simulink library "EV_VLD"  (R2019b)
settings: Solver=VariableStepAuto  StartTime=0.0  StopTime=10.0  RelTol=1e-3
undefined symbols (not defined in the file): DiscIntNeverNeededParam
libraries: $bdroot x2, simulink x2
(part 1 of 2)
Description:
  | User defined library for EV
settings Model: Creator=francesco.mantuano  LastModifiedBy=francesco.mantuano

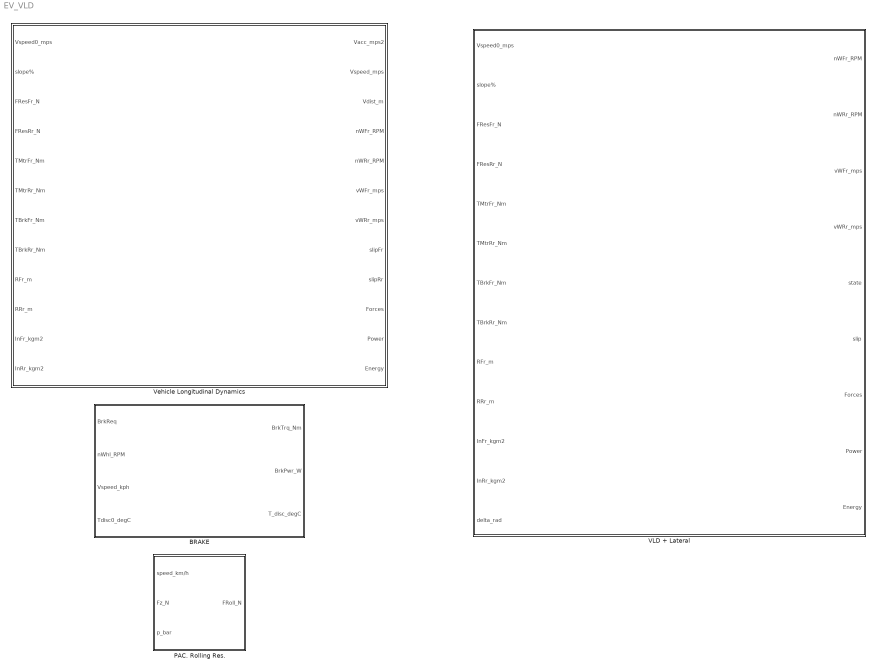
== system EV_VLD ==
  BRAKE : Subsystem  mask(Brake){MxTrq_Nm=7200, eff=1, HC_disc=3420, T_env_degC=0, R_StoC_KpW=0.0035*0.8, HTC_v_bp=0:150:300, HTC_map=[3 20 40]}
      mask prompts: MxTrq_Nm "Max torque [Nm]"; eff "Efficiency"; HC_disc "HC_disc [J/K]"; T_env_degC "T_env [°C]"; R_StoC_KpW "R_StoC [K/W]"; HTC_v_bp "Speed [km/h] bp"; HTC_map "HTC [W/K]"
      mask help: The BRAKE block gives as outputs the brake torque and the thrmal power dissipated. It also estimates the brake discs temperature.
      mask DialogControl Container2 Prompt: Inputs description
      mask DialogControl DescTextVar Prompt: - BrkReq: brake requested from VCU (0 < BrkReq < 1) [-]
      mask DialogControl Control4 Prompt: - nWhl_RPM: wheels speed [RPM]
      mask DialogControl Control5 Prompt: - Vspeed_mps: vehicle speed [m/s]
      mask DialogControl Control6 Prompt: - Tbrake0_degC: initial temperature of the brake discs [°C]
      mask DialogControl Container3 Prompt: Parameters
      mask DialogControl Container9 Prompt: Mechanical
      mask DialogControl Container5 Prompt: Thermal
      mask DialogControl Container10 Prompt: HTC map
  PAC. Rolling Res. : Subsystem  mask(Rolling Resistance (Pacejka)){Vref_kmph=130, Fzref_N=5540, pref_bar=3, SF=1.15, qsy1=8.37e-3, qsy2=0, qsy3=1.02e-3, qsy4=-2.51e-5, qsy5=0, qsy6=0, qsy7=0.865, qsy8=-0.337}
      mask prompts: Vref_kmph "Vref [km/h]"; Fzref_N "Fzref [N]"; pref_bar "pref [bar]"; SF "scaling factor"
      mask help: Pacejka rolling resistance force calculation (one tire)
  VLD + Lateral : Subsystem  mask(Vehicle Longitudinal Dynamics){mass_kg=2000, J_kgm2=3000, WDFr_p=48, l_m=2.800, t1=1.765, t2=1.725, hCOG_m=0.45, h1=0.15, h2=0.18, q=0.285, k1=1e5, k2=1.2e5, Tenv_degC=23, Fsurf_sm=2.4, Cl_Fr1=0, Cl_Rr1=0, Cd1=0.35, WRS_kmph=160, Cl_Fr2=-0.1, Cl_Rr2=-0.2, Cd2=0.4, VLoad_bp=0, slip_bp=0, frictionFr_map=0, frictionRr_map=0, VLoada_bp=0, slipa_bp=0, FyFr_map=0, FyRr_map=0}
      mask prompts: mass_kg "Mass [kg]"; J_kgm2 "Yaw Inertia [kg*sm]"; WDFr_p "Weight distribution Front [%]"; l_m "Vehicle wheelbase [m]"; t1 "Front track [m]"; t2 "Rear track [m]"; hCOG_m "COG height [m]"; h1 "Front Roll center height [m]"; h2 "Rear Roll center height [m]"; q "COG-RollAxle distance [m]"; k1 "Front Roll stiffness [Nm/rad]"; k2 "Rear Roll stiffness [Nm/rad]"; Tenv_degC "Ambient temperature [degC]"; Fsurf_sm "Frontal area [sm]"; Cl_Fr1 "Lift coefficient FRONT"; Cl_Rr1 "Lift coefficient REAR"; Cd1 "Drag coefficient"; WRS_kmph "Wing Raise Speed [km/h]"; Cl_Fr2 "Lift coefficient FRONT"; Cl_Rr2 "Lift coefficient REAR"; Cd2 "Drag coefficient"; VLoad_bp "Vertical Load [N] breakpoints"; slip_bp "longitudinal slip [-] breakpoints"; frictionFr_map "Front friction coefficient MAP"; frictionRr_map "Rear friction coefficient MAP"; VLoada_bp "Vertical Load [N] breakpoints"; slipa_bp "lateral slip [rad] breakpoints"; FyFr_map "Front friction coefficient MAP"; FyRr_map "Rear friction coefficient MAP"
      mask help:
      | The VLD block is an estimation block that calculate the Vehicle state. It also outputs the Forces, the Power and the Energy involved.
      | NOTE THAT: the motor torque is already delayed in the estimation block.
      mask DialogControl Container2 Prompt: Inputs description
      mask DialogControl DescTextVar Prompt: - Vspeed0_mps: initial speed of the vehicle [m/s]
      mask DialogControl Control4 Prompt: - slope%: inclination of the road [%]
      mask DialogControl Control5 Prompt: - FResFr_N: front resistance force acting before the tires [N]
      mask DialogControl Control6 Prompt: - FResRr_N: rear resistance force acting before the tires [N]
      mask DialogControl Control8 Prompt: - TMtrFr_Nm: front motor torque [Nm]
      mask DialogControl Control9 Prompt: - TMtrRr_Nm: rear motor torque [Nm]
      mask DialogControl Control10 Prompt: - TBrkFr_Nm: front brake torque [Nm]
      mask DialogControl Control11 Prompt: - TBrkRr_Nm: rear brake torque [Nm]
      mask DialogControl Control12 Prompt: - RFr_m: front rolling radius [m]
      mask DialogControl Control13 Prompt: - RRr_m: rear rolling radius [m]
      mask DialogControl Control14 Prompt: - InFr_kgm2: front rotational inertia [kg*sm]
      mask DialogControl Control15 Prompt: - InRr_kgm2: rear rotational inertia [kg*sm]
      mask DialogControl Container11 Prompt: Outputs description
      mask DialogControl Control16 Prompt: - Vacc_mps2: vehicle acceleration [m/s2]
      mask DialogControl Control17 Prompt: - Vspeed_mps: vehicle speed [m/s]
      mask DialogControl Control18 Prompt: - Vdist_m: distance traveled [m]
      mask DialogControl Control19 Prompt: - nWFr_RPM: front wheels RPM
      mask DialogControl Control20 Prompt: - nWRr_RPM: rear wheels RPM
      mask DialogControl Control21 Prompt: - vWFr_mps: front wheels speed [m/s]
      mask DialogControl Control22 Prompt: - vWRr_mps: rear wheels speed [m/s]
      mask DialogControl Control23 Prompt: - slipFr: front tires longitudinal slip [-]
      mask DialogControl Control24 Prompt: - slipRr: rear tires longitudinal slip [-]
      mask DialogControl Container12 Prompt: Forces
      mask DialogControl Control25 Prompt: - mequiv_kg: vehicle equivalent mass [kg]
      mask DialogControl Control26 Prompt: - WFr_N: front vertical load [N]
      mask DialogControl Control27 Prompt: - WRr_N: rear vertical load [N]
      mask DialogControl Control28 Prompt: - FWhl_N: total traction force (includes braking force) [N]
      mask DialogControl Control29 Prompt: - FResTot_N: total resistance force [N]
      mask DialogControl Control30 Prompt: - FTot_N: FWhl - FResTot [N]
      mask DialogControl Container14 Prompt: Power
      mask DialogControl Control31 Prompt: - PWhl_W: traction power (includes brake) at wheels [W]
      mask DialogControl Control32 Prompt: - PWhlMtr_W: motor traction power at wheels [W]
      mask DialogControl Container13 Prompt: Energy
      mask DialogControl Control33 Prompt: - EWhlMtrC_kWh: motor charge energy at wheels [kWh]
      mask DialogControl Control34 Prompt: - EWhlMtrD_kWh: motor discharge energy at wheels [kWh]
      mask DialogControl Control35 Prompt: - EDrag_kWh: drag energy loss [kWh]
      mask DialogControl Container3 Prompt: Vehicle parameters
      mask DialogControl Container9 Prompt: Weights
      mask DialogControl Container5_copy Prompt: Aerodynamics
      mask DialogControl Container10 Prompt: Active Wing
      mask DialogControl Container5 Prompt: Tire
      mask DialogControl Container17 Prompt: Longitudinal
      mask DialogControl Container17_copy Prompt: Lateral
  Vehicle Longitudinal Dynamics : Subsystem  mask(Vehicle Longitudinal Dynamics){slip=0, mass_kg=2000, WDFr_p=48, l_m=2.800, hCOG_m=0.45, tow_mass_kg=0, h_tow=0.5, Tenv_degC=23, Fsurf_sm=2.4, Cl_Fr1=0, Cl_Rr1=0, Cd1=0, WRS_kmph=0, Cl_Fr2=0, Cl_Rr2=0, Cd2=0, VLoad_bp=zeros(1,2), slip_bp=zeros(1,2), frictionFr_map=zeros(2,2), frictionRr_map=zeros(2,2), mu_front=0.8, mu_rear=0.8}
      mask prompts: slip "slip (== 1 slip model, == 0 no-slip model)"; mass_kg "Mass [kg]"; WDFr_p "Weight distribution Front [%]"; l_m "Vehicle wheelbase [m]"; hCOG_m "COG height [m]"; tow_mass_kg "Mass [kg]"; h_tow "Hitch height [m]"; Tenv_degC "Ambient temperature [degC]"; Fsurf_sm "Frontal area [sm]"; Cl_Fr1 "Lift coefficient FRONT"; Cl_Rr1 "Lift coefficient REAR"; Cd1 "Drag coefficient"; WRS_kmph "Wing Raise Speed [km/h]"; Cl_Fr2 "Lift coefficient FRONT"; Cl_Rr2 "Lift coefficient REAR"; Cd2 "Drag coefficient"; VLoad_bp "Vertical Load [N] breakpoints"; slip_bp "longitudinal slip [-] breakpoints"; frictionFr_map "Front friction coefficient MAP"; frictionRr_map "Rear friction coefficient MAP"; mu_front "front mu [-]"; mu_rear "rear mu [-]"
      mask help:
      | The VLD block is an estimation block that calculate the Vehicle state. It also outputs the Forces, the Power and the Energy involved.
      | NOTE THAT: the motor torque is already delayed in the estimation block.
      mask DialogControl Container2 Prompt: Inputs description
      mask DialogControl DescTextVar Prompt: - Vspeed0_mps: initial speed of the vehicle [m/s]
      mask DialogControl Control4 Prompt: - slope%: inclination of the road [%]
      mask DialogControl Control5 Prompt: - FResFr_N: front resistance force acting before the tires [N]
      mask DialogControl Control6 Prompt: - FResRr_N: rear resistance force acting before the tires [N]
      mask DialogControl Control8 Prompt: - TMtrFr_Nm: front motor torque [Nm]
      mask DialogControl Control9 Prompt: - TMtrRr_Nm: rear motor torque [Nm]
      mask DialogControl Control10 Prompt: - TBrkFr_Nm: front brake torque [Nm]
      mask DialogControl Control11 Prompt: - TBrkRr_Nm: rear brake torque [Nm]
      mask DialogControl Control12 Prompt: - RFr_m: front rolling radius [m]
      mask DialogControl Control13 Prompt: - RRr_m: rear rolling radius [m]
      mask DialogControl Control14 Prompt: - InFr_kgm2: front rotational inertia [kg*sm]
      mask DialogControl Control15 Prompt: - InRr_kgm2: rear rotational inertia [kg*sm]
      mask DialogControl Container11 Prompt: Outputs description
      mask DialogControl Control16 Prompt: - Vacc_mps2: vehicle acceleration [m/s2]
      mask DialogControl Control17 Prompt: - Vspeed_mps: vehicle speed [m/s]
      mask DialogControl Control18 Prompt: - Vdist_m: distance traveled [m]
      mask DialogControl Control19 Prompt: - nWFr_RPM: front wheels RPM
      mask DialogControl Control20 Prompt: - nWRr_RPM: rear wheels RPM
      mask DialogControl Control21 Prompt: - vWFr_mps: front wheels speed [m/s]
      mask DialogControl Control22 Prompt: - vWRr_mps: rear wheels speed [m/s]
      mask DialogControl Control23 Prompt: - slipFr: front tires longitudinal slip [-]
      mask DialogControl Control24 Prompt: - slipRr: rear tires longitudinal slip [-]
      mask DialogControl Container12 Prompt: Forces
      mask DialogControl Control25 Prompt: - mequiv_kg: vehicle equivalent mass [kg]
      mask DialogControl Control26 Prompt: - WFr_N: front vertical load [N]
      mask DialogControl Control27 Prompt: - WRr_N: rear vertical load [N]
      mask DialogControl Control28 Prompt: - FWhl_N: total traction force (includes braking force) [N]
      mask DialogControl Control29 Prompt: - FResTot_N: total resistance force [N]
      mask DialogControl Control30 Prompt: - FTot_N: FWhl - FResTot [N]
      mask DialogControl Container14 Prompt: Power
      mask DialogControl Control31 Prompt: - PWhl_W: traction power (includes brake) at wheels [W]
      mask DialogControl Control32 Prompt: - PWhlMtr_W: motor traction power at wheels [W]
      mask DialogControl Container13 Prompt: Energy
      mask DialogControl Control33 Prompt: - EWhlMtrC_kWh: motor charge energy at wheels [kWh]
      mask DialogControl Control34 Prompt: - EWhlMtrD_kWh: motor discharge energy at wheels [kWh]
      mask DialogControl Control35 Prompt: - EDrag_kWh: drag energy loss [kWh]
      mask DialogControl Container3 Prompt: Vehicle parameters
      mask DialogControl Container9 Prompt: Weights
      mask DialogControl Container19 Prompt: Towing
      mask DialogControl Container5_copy Prompt: Aerodynamics
      mask DialogControl Container10 Prompt: Active Wing
      mask DialogControl Container5 Prompt: Tire
      mask DialogControl Container17 Prompt: slip model
      mask DialogControl Container18 Prompt: no-slip model

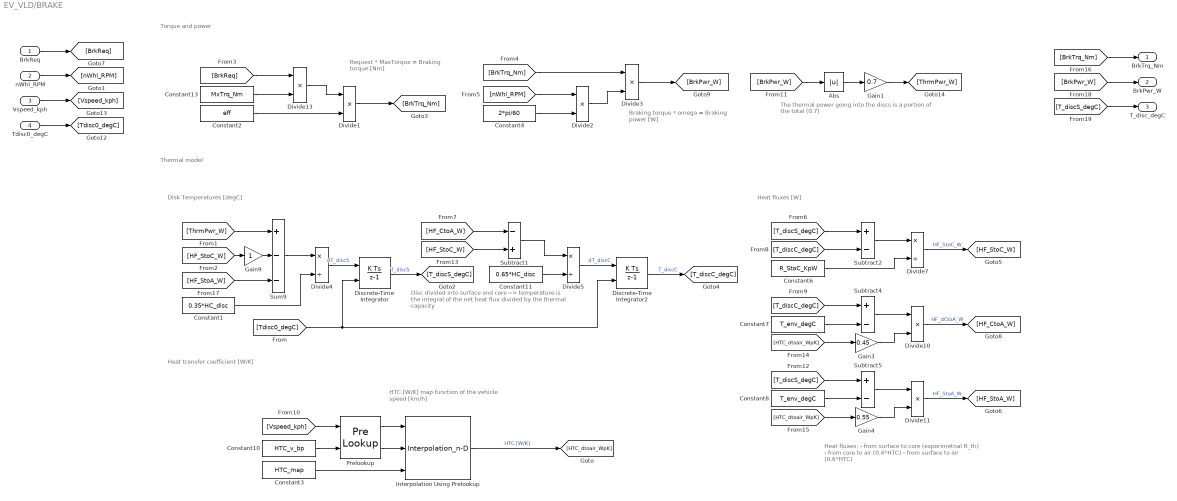
== system EV_VLD/BRAKE ==
  note: Torque and power
  note: Thermal model
  note: The thermal power going into the discs is a portion of the total (0.7)
  note: Request * MaxTorque = Braking torque [Nm]
  note: Heat fluxes [W]
  note: Disk Temperatures [degC]
  note: Braking torque * omega = Braking power [W]
  note: Heat transfer coefficient [W/K]
  note: HTC [W/K] map function of the vehicle speed [km/h]
  note: Heat fluxes:
      | - from surface to core (experimetnal R_th)
      | - from core to air (0.4*HTC)
      | - from surface to air (0.6*HTC)
  note: Disc divided into surface and core --> temperature is the integral of the net heat flux divided by the thermal capacity
  BrkReq : Inport
  nWhl_RPM : Inport  Port=2
  Vspeed_kph : Inport  Port=3
  Tdisc0_degC : Inport  Port=4
  Abs : Abs
  Constant1 : Constant  Value=0.35*HC_disc
  Constant10 : Constant  Value=HTC_v_bp
  Constant11 : Constant  Value=0.65*HC_disc
  Constant13 : Constant  Value=MxTrq_Nm
  Constant2 : Constant  Value=eff
  Constant3 : Constant  Value=HTC_map
  Constant4 : Constant  Value=2*pi/60
  Constant6 : Constant  Value=R_StoC_KpW
  Constant7 : Constant  Value=T_env_degC
  Constant8 : Constant  Value=T_env_degC
  Discrete-Time Integrator : DiscreteIntegrator  InitialConditionSource=external  SampleTime=-1  ICPrevOutput=DiscIntNeverNeededParam  ICPrevScaledInput=DiscIntNeverNeededParam
  Discrete-Time Integrator2 : DiscreteIntegrator  InitialConditionSource=external  SampleTime=-1  ICPrevOutput=DiscIntNeverNeededParam  ICPrevScaledInput=DiscIntNeverNeededParam
  Divide{1..3,13} (4 alike) : Product
  Divide10 : Product  Inputs=**
  Divide11 : Product  Inputs=**
  Divide4 : Product  Inputs=*/
  Divide5 : Product  Inputs=*/
  Divide7 : Product  Inputs=*/
  Gain1 : Gain  Gain=0.7
  Gain3 : Gain  Gain=0.45
  Gain4 : Gain  Gain=0.55
  Gain9 : Gain
  Interpolation Using Prelookup : Interpolation_n-D  NumberOfTableDimensions=1  TableSource=Input port  InternalRulePriority=Speed
      settings: InputPortMap=u0,u1,p2
  Prelookup : PreLookup  BreakpointsDataSource=Input port  BreakpointsData=[10:10:110]  ExtrapMethod=Linear
      settings: InputPortMap=u0,p1
  Subtract1 : Sum  Inputs=-+
  Subtract2 : Sum  Inputs=+-
  Subtract4 : Sum  Inputs=+-
  Subtract5 : Sum  Inputs=+-
  Sum9 : Sum  Inputs=+--
  BrkTrq_Nm : Outport
  BrkPwr_W : Outport  Port=2
  T_disc_degC : Outport  Port=3
  wires:
  nWhl_RPM/1 -> [nWhl_RPM]
  BrkReq/1 -> [BrkReq]
  Gain9/1 -> Sum9/2
  [ThrmPwr_W] -> Sum9/1
  Constant6/1 -> Divide7/2
  Constant1/1 -> Divide4/2
  Sum9/1 -> Divide4/1
  Discrete-Time Integrator/1 -> [T_discS_degC]  "T_discS"
  Discrete-Time Integrator2/1 -> [T_discC_degC]  "T_discC"
  Divide5/1 -> Discrete-Time Integrator2/1  "dT_discC"
  Divide4/1 -> Discrete-Time Integrator/1  "dT_discS"
  [Tdisc0_degC] -> Discrete-Time Integrator/2, Discrete-Time Integrator2/2
  [HF_StoC_W] -> Gain9/1
  Divide7/1 -> [HF_StoC_W]  "HF_StoC_W"
  [HF_StoA_W] -> Sum9/3
  Vspeed_kph/1 -> [Vspeed_kph]
  Tdisc0_degC/1 -> [Tdisc0_degC]
  [BrkReq] -> Divide13/1
  Constant13/1 -> Divide13/2
  Divide13/1 -> Divide1/1
  Constant2/1 -> Divide1/2
  Divide1/1 -> [BrkTrq_Nm]
  [nWhl_RPM] -> Divide2/1
  Constant4/1 -> Divide2/2
  [BrkTrq_Nm] -> Divide3/1
  Divide2/1 -> Divide3/2
  Divide3/1 -> [BrkPwr_W]
  [BrkPwr_W] -> Abs/1
  Gain1/1 -> [ThrmPwr_W]
  [HF_StoC_W] -> Subtract1/2
  [HF_CtoA_W] -> Subtract1/1
  Subtract1/1 -> Divide5/1
  Constant11/1 -> Divide5/2
  Interpolation Using Prelookup/1 -> [HTC_dtoair_WpK]  "HTC [W/K]"
  [T_discS_degC] -> Subtract2/1
  [T_discC_degC] -> Subtract2/2
  Subtract2/1 -> Divide7/1
  Subtract4/1 -> Divide10/1
  Constant7/1 -> Subtract4/2
  [T_discC_degC] -> Subtract4/1
  Divide10/1 -> [HF_CtoA_W]  "HF_dCtoA_W"
  [HTC_dtoair_WpK] -> Gain3/1
  [HTC_dtoair_WpK] -> Gain4/1
  Divide11/1 -> [HF_StoA_W]  "HF_StoA_W"
  [T_discS_degC] -> Subtract5/1
  Constant8/1 -> Subtract5/2
  Subtract5/1 -> Divide11/1
  Gain3/1 -> Divide10/2
  Gain4/1 -> Divide11/2
  [BrkTrq_Nm] -> BrkTrq_Nm/1
  [BrkPwr_W] -> BrkPwr_W/1
  [T_discS_degC] -> T_disc_degC/1
  Abs/1 -> Gain1/1
  Prelookup/1 -> Interpolation Using Prelookup/1
  Prelookup/2 -> Interpolation Using Prelookup/2
  Constant10/1 -> Prelookup/2
  Constant3/1 -> Interpolation Using Prelookup/3
  [Vspeed_kph] -> Prelookup/1

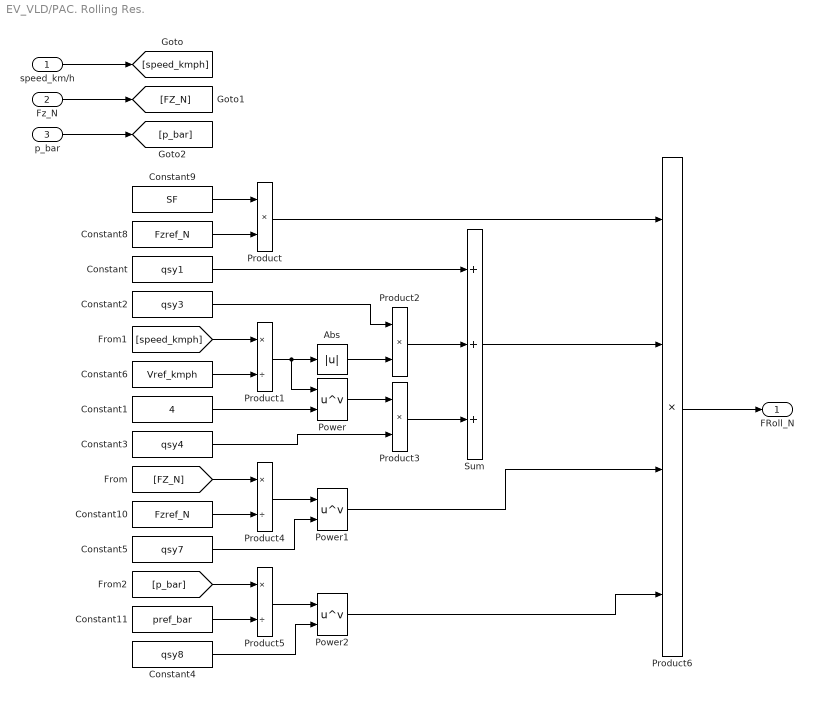
== system EV_VLD/PAC. Rolling Res. ==
  speed_km/h : Inport
  Fz_N : Inport  Port=2
  p_bar : Inport  Port=3
  Abs : Abs
  Constant : Constant  Value=qsy1
  Constant1 : Constant  Value=4
  Constant10 : Constant  Value=Fzref_N
  Constant11 : Constant  Value=pref_bar
  Constant2 : Constant  Value=qsy3
  Constant3 : Constant  Value=qsy4
  Constant4 : Constant  Value=qsy8
  Constant5 : Constant  Value=qsy7
  Constant6 : Constant  Value=Vref_kmph
  Constant8 : Constant  Value=Fzref_N
  Constant9 : Constant  Value=SF
  Power : Math  Operator=pow  SignedPower=off  SaturateOnIntegerOverflow=on
  Power1 : Math  Operator=pow  SignedPower=off  SaturateOnIntegerOverflow=on
  Power2 : Math  Operator=pow  SignedPower=off  SaturateOnIntegerOverflow=on
  Product : Product
  Product1 : Product  Inputs=*/
  Product2 : Product
  Product3 : Product
  Product4 : Product  Inputs=*/
  Product5 : Product  Inputs=*/
  Product6 : Product  Inputs=4
  Sum : Sum  Inputs=+++
  FRoll_N : Outport
  wires:
  Constant9/1 -> Product/1
  Constant8/1 -> Product/2
  speed_km/h/1 -> [speed_kmph]
  Constant6/1 -> Product1/2
  [speed_kmph] -> Product1/1
  Product1/1 -> Power/1, Abs/1
  Constant2/1 -> Product2/1
  Abs/1 -> Product2/2
  Constant1/1 -> Power/2
  Power/1 -> Product3/1
  Constant3/1 -> Product3/2
  Constant/1 -> Sum/1
  Product3/1 -> Sum/3
  Product2/1 -> Sum/2
  Fz_N/1 -> [FZ_N]
  [FZ_N] -> Product4/1
  Constant10/1 -> Product4/2
  Product4/1 -> Power1/1
  Constant5/1 -> Power1/2
  [p_bar] -> Product5/1
  Constant11/1 -> Product5/2
  Product5/1 -> Power2/1
  Constant4/1 -> Power2/2
  Power2/1 -> Product6/4
  Power1/1 -> Product6/3
  Sum/1 -> Product6/2
  Product/1 -> Product6/1
  Product6/1 -> FRoll_N/1
  p_bar/1 -> [p_bar]

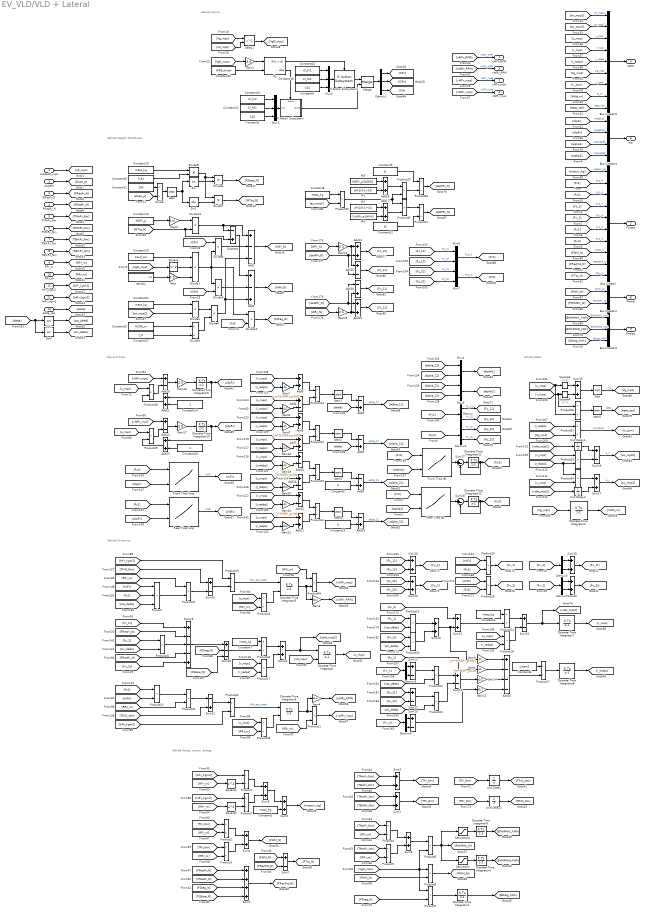
== system EV_VLD/VLD + Lateral ==
  note: Vehicle forces, power, energy
  note: Vehicle Weight Distribution
  note: Slip and Tires
  note: Vehicle Dynamics
  note: Aerodynamics
  note: Vehicle State
  Vspeed0_mps : Inport
  slope% : Inport  Port=2
  FResFr_N : Inport  Port=3
  FResRr_N : Inport  Port=4
  TMtrFr_Nm : Inport  Port=5
  TMtrRr_Nm : Inport  Port=6
  TBrkFr_Nm : Inport  Port=7
  TBrkRr_Nm : Inport  Port=8
  RFr_m : Inport  Port=9
  RRr_m : Inport  Port=10
  InFr_kgm2 : Inport  Port=11
  InRr_kgm2 : Inport  Port=12
  delta_rad : Inport  Port=13
  Add1 : Sum  Inputs=+-+
  Add{4,10,12,15,19,22,24} (7 alike) : Sum  Inputs=+-
  Add{6..8,11,13..14,17..18,21,23} (10 alike) : Sum
  Add{3,5,9,16,25} (5 alike) : Sum  Inputs=-+
  Add2 : Sum  Inputs=+--
  Add20 : Sum  Inputs=+---
  Atan{,1..5} (6 alike) : Trigonometry  Operator=atan
  Bus Creator : BusCreator  Inputs=10
  Bus Creator2 : BusCreator  Inputs=2
  Bus Creator3 : BusCreator  Inputs=3
  Bus Creator4 : BusCreator  Inputs=4
  Bus Creator5 : BusCreator  Inputs=9
  Constant{1,3,7..8,19,22} (6 alike) : Constant  Value=mass_kg
  Constant10 : Constant  Value=Fsurf_sm
  Constant11 : Constant  Value=Cl_Rr2
  Constant12 : Constant  Value=t2
  Constant13 : Constant  Value=WDFr_p
  Constant14 : Constant
  Constant15 : Constant  Value=hCOG_m
  Constant16 : Constant  Value=9.81
  Constant17 : Constant  Value=l_m
  Constant18 : Constant  Value=Cl_Rr1
  Constant2 : Constant  Value=Cd2
  Constant20 : Constant  Value=Cl_Fr2
  Constant21 : Constant  Value=100
  Constant23 : Constant  Value=WRS_kmph
  Constant24 : Constant  Value=Cl_Fr1
  Constant25 : Constant  Value=0
  Constant26 : Constant
  Constant4 : Constant  Value=Cd1
  Constant5 : Constant  Value=0
  Constant6 : Constant  Value=J_kgm2
  Constant9 : Constant  Value=t1
  Delay1 : Delay  DelayLength=1  InitialConditionSource=Input port
      settings: InputPortMap=u0,p4
  Demux{,2..6} (6 alike) : Demux  Outputs=2
  Demux1 : Demux  Outputs=3
  Discrete-Time Integrator : DiscreteIntegrator  InitialConditionSource=external  SampleTime=-1  LimitOutput=on  LowerSaturationLimit=1e-6  ICPrevOutput=DiscIntNeverNeededParam  ICPrevScaledInput=DiscIntNeverNeededParam
  Discrete-Time Integrator1 : DiscreteIntegrator  gainval=1e-3/3600  SampleTime=-1  ICPrevOutput=DiscIntNeverNeededParam  ICPrevScaledInput=DiscIntNeverNeededParam
  Discrete-Time Integrator10 : DiscreteIntegrator  gainval=1  SampleTime=-1  LimitOutput=on  UpperSaturationLimit=1  LowerSaturationLimit=-1  ICPrevOutput=DiscIntNeverNeededParam  ICPrevScaledInput=DiscIntNeverNeededParam
  Discrete-Time Integrator11 : DiscreteIntegrator  gainval=1/0.055  SampleTime=-1  ICPrevOutput=DiscIntNeverNeededParam  ICPrevScaledInput=DiscIntNeverNeededParam
  Discrete-Time Integrator12 : DiscreteIntegrator  gainval=1/0.055  SampleTime=-1  ICPrevOutput=DiscIntNeverNeededParam  ICPrevScaledInput=DiscIntNeverNeededParam
  Discrete-Time Integrator2 : DiscreteIntegrator  SampleTime=-1  LowerSaturationLimit=0  ICPrevOutput=DiscIntNeverNeededParam  ICPrevScaledInput=DiscIntNeverNeededParam
  Discrete-Time Integrator3 : DiscreteIntegrator  InitialConditionSource=external  SampleTime=-1  LimitOutput=on  LowerSaturationLimit=0  ICPrevOutput=DiscIntNeverNeededParam  ICPrevScaledInput=DiscIntNeverNeededParam
  Discrete-Time Integrator4 : DiscreteIntegrator  gainval=1e-3/3600  SampleTime=-1  ICPrevOutput=DiscIntNeverNeededParam  ICPrevScaledInput=DiscIntNeverNeededParam
  Discrete-Time Integrator5 : DiscreteIntegrator  gainval=1e-3/3600  SampleTime=-1  ICPrevOutput=DiscIntNeverNeededParam  ICPrevScaledInput=DiscIntNeverNeededParam
  Discrete-Time Integrator6 : DiscreteIntegrator  InitialConditionSource=external  SampleTime=-1  LimitOutput=on  LowerSaturationLimit=0  ICPrevOutput=DiscIntNeverNeededParam  ICPrevScaledInput=DiscIntNeverNeededParam
  Discrete-Time Integrator7 : DiscreteIntegrator  SampleTime=-1  ICPrevOutput=DiscIntNeverNeededParam  ICPrevScaledInput=DiscIntNeverNeededParam
  Discrete-Time Integrator8 : DiscreteIntegrator  SampleTime=-1  ICPrevOutput=DiscIntNeverNeededParam  ICPrevScaledInput=DiscIntNeverNeededParam
  Discrete-Time Integrator9 : DiscreteIntegrator  gainval=1  SampleTime=-1  LimitOutput=on  UpperSaturationLimit=1  LowerSaturationLimit=-1  ICPrevOutput=DiscIntNeverNeededParam  ICPrevScaledInput=DiscIntNeverNeededParam
  Divide : Product  Inputs=/*
  Divide1 : Product  Inputs=***
  Divide{2,4..10,13} (9 alike) : Product
  Divide3 : Product  Inputs=*/
  Front Tires lat : Lookup_n-D  BreakpointsForDimension1=VLoada_bp  BreakpointsForDimension2=slipa_bp  Table=FyFr_map  InternalRulePriority=Speed  RndMeth=Simplest  InputSameDT=on
  Front Tires long : Lookup_n-D  BreakpointsForDimension1=VLoad_bp  BreakpointsForDimension2=slip_bp  Table=frictionFr_map  InternalRulePriority=Speed  RndMeth=Simplest  InputSameDT=on
  Gain : Gain  Gain=0.5
  Gain1 : Gain  Gain=3.6
  Gain10 : Gain  Gain=l_m*WDFr_p/100
  Gain11 : Gain  Gain=t2/2
  Gain12 : Gain  Gain=0.5
  Gain13 : Gain  Gain=t2/2
  Gain14 : Gain  Gain=t1/2
  Gain15 : Gain  Gain=0.5
  Gain16 : Gain  Gain=2.5
  Gain17 : Gain  Gain=2.5
  Gain18 : Gain  Gain=t1/2
  Gain19 : Gain  Gain=l_m*WDFr_p/100
  Gain2 : Gain  Gain=0.01
  Gain20 : Gain  Gain=t2/2
  Gain3 : Gain  Gain=30/pi
  Gain4 : Gain  Gain=30/pi
  Gain5 : Gain  Gain=l_m*(1-WDFr_p/100)
  Gain6 : Gain  Gain=l_m*WDFr_p/100
  Gain7 : Gain  Gain=l_m*(1-WDFr_p/100)
  Gain8 : Gain  Gain=t1/2
  Gain9 : Gain  Gain=l_m*(1-WDFr_p/100)
  If Action Subsystem : Subsystem  TreatAsAtomicUnit=on
  If Action Subsystem1 : $bdroot/Vehicle Longitudinal Dynamics/If Action Subsystem  SystemSampleTime=-1  Latency=0  AutoFrameSizeCalculation=off
  If1 : If  NumInputs=2  IfExpression=u1 < u2
  M1 : Constant  Value=q*k1/(k1+k2)
  M2 : Constant  Value=q*k2/(k1+k2)
  M3 : Constant  Value=WDFr_p/100*h2
  M4 : Constant  Value=(1-WDFr_p/100)*h2
  Merge : Merge
  Mux1 : Mux  Inputs=3
  Mux3 : Mux  Inputs=3
  Mux{4..7} (4 alike) : Mux  Inputs=2
  Product : Product  Inputs=***
  Product{1..5,7,12..15,28,31,37,41,43..44} (16 alike) : Product  Inputs=*/
  Product{10..11,16..23,25..26,29..30,32,35,45} (17 alike) : Product
  Product{24,27,36,40,42} (5 alike) : Product  Inputs=/*
  Product{6,8..9,33..34,38..39} (7 alike) : Product  Inputs=**
  Rear Tires lat : Lookup_n-D  BreakpointsForDimension1=VLoada_bp  BreakpointsForDimension2=slipa_bp  Table=FyFr_map  InternalRulePriority=Speed  RndMeth=Simplest  InputSameDT=on
  Rear Tires long : Lookup_n-D  BreakpointsForDimension1=VLoad_bp  BreakpointsForDimension2=slip_bp  Table=frictionRr_map  InternalRulePriority=Speed  RndMeth=Simplest  InputSameDT=on
  Saturation : Saturate  UpperLimit=inf  LowerLimit=0
  Saturation1 : Saturate  UpperLimit=0  LowerLimit=-inf
  Sin : Trigonometry
  Sin1 : Trigonometry  Operator=cos
  Sin2 : Trigonometry  Operator=cos
  Sin3 : Trigonometry
  Sqrt : Sqrt  SaturateOnIntegerOverflow=on
  Square : Math  Operator=square  SignedPower=off  SaturateOnIntegerOverflow=on
  Square1 : Math  Operator=square  SignedPower=off  SaturateOnIntegerOverflow=on
  Square2 : Math  Operator=square  SignedPower=off  SaturateOnIntegerOverflow=on
  Square3 : Math  Operator=square  SaturateOnIntegerOverflow=on
  Square4 : Math  Operator=square  SaturateOnIntegerOverflow=on
  Subtract : Sum  Inputs=-+
  Sum1 : Sum  Inputs=++++
  Sum{2..6,8,10..11,16..17,24..26,29..30} (15 alike) : Sum
  Sum{7,12..15,18,22..23} (8 alike) : Sum  Inputs=+-
  Sum19 : Sum  Inputs=+---+
  Sum20 : Sum  Inputs=+--
  Sum21 : Sum  Inputs=-+
  Sum27 : Sum  Inputs=|+-
  Sum28 : Sum  Inputs=|+-
  Unit Delay{,1..3} (4 alike) : UnitDelay  SampleTime=-1  HasFrameUpgradeWarning=on
  density : Subsystem
  nWFr_RPM : Outport
  nWRr_RPM : Outport  Port=2
  vWFr_mps : Outport  Port=3
  vWRr_mps : Outport  Port=4
  state : Outport  Port=5
  slip : Outport  Port=6
  Forces : Outport  Port=7
  Power : Outport  Port=8
  Energy : Outport  Port=9
  wires:
  [EDrag_kWh] -> Bus Creator3/3  "EDrag_kWh"
  Discrete-Time Integrator1/1 -> [EDrag_kWh]
  Product9/1 -> Discrete-Time Integrator1/1
  [FDrag_N] -> Product9/2
  Divide10/1 -> [FDrag_N]
  [Cd] -> Divide10/2
  Constant2/1 -> Mux1/3
  Constant11/1 -> Mux1/2
  Constant20/1 -> Mux1/1
  Demux1/3 -> [Cd]
  Constant4/1 -> Mux3/3
  Unit Delay2/1 -> [TRrD_Nm]
  Unit Delay/1 -> [TFrD_Nm]
  [TRr_Nm] -> Unit Delay2/1
  [TFr_Nm] -> Unit Delay/1
  Bus Creator3/1 -> Energy/1
  [EWhlMtrC_kWh] -> Bus Creator3/1  "EWhlMtrC_kWh"
  [EWhlMtrD_kWh] -> Bus Creator3/2  "EWhlMtrD_kWh"
  [PWhlMtr_W] -> Bus Creator2/2  "PWhlMtr_W"
  [PWhl_W] -> Bus Creator2/1  "PWhl_W"
  Saturation/1 -> Discrete-Time Integrator4/1
  Saturation1/1 -> Discrete-Time Integrator5/1
  Discrete-Time Integrator4/1 -> [EWhlMtrD_kWh]
  Discrete-Time Integrator5/1 -> [EWhlMtrC_kWh]
  Product8/1 -> [PWhl_W]
  [FWhl_N] -> Product8/2
  Product6/1 -> [PWhlMtr_W], Saturation/1, Saturation1/1
  [VgD_mps] -> Product6/2, Product8/1, Product9/1
  Sum8/1 -> Product6/1
  [RRr_m] -> Product5/2
  [RFr_m] -> Product4/2
  [TMtrFr_Nm] -> Product4/1
  Product5/1 -> Sum8/2
  [TMtrRr_Nm] -> Product5/1
  Product4/1 -> Sum8/1
  Bus Creator2/1 -> Power/1
  [FTot_N] -> Bus Creator/10  "FTot_N"
  Sum7/1 -> [FTot_N]
  [FResTot_N] -> Sum7/2
  [FWhl_N] -> Sum7/1
  [TMtrRr_Nm] -> Sum2/1
  [TBrkRr_Nm] -> Sum2/2
  Sum2/1 -> [TRr_Nm]
  [TBrkFr_Nm] -> Sum3/2
  [TMtrFr_Nm] -> Sum3/1
  Sum3/1 -> [TFr_Nm]
  TBrkRr_Nm/1 -> [TBrkRr_Nm]
  TBrkFr_Nm/1 -> [TBrkFr_Nm]
  Bus Creator/1 -> Forces/1
  [FResTot_N] -> Bus Creator/9  "FResTot_N"
  [FWhl_N] -> Bus Creator/8  "FWhl_N"
  [mequiv_kg] -> Bus Creator/1  "mequiv_kg"
  [FSlope_N] -> Sum1/4
  Product2/1 -> Sum4/1
  Sum6/1 -> Sum5/1
  Square1/1 -> Product1/2
  [TRr_Nm] -> Product3/1
  Sum1/1 -> [FResTot_N]
  Constant1/1 -> Sum5/2
  Product3/1 -> Sum4/2
  [TFr_Nm] -> Product2/1
  [RFr_m] -> Product2/2
  Square2/1 -> Product7/2
  Sum4/1 -> [FWhl_N]
  [RRr_m] -> Product3/2
  Product1/1 -> Sum6/1
  [FResFr_N] -> Sum1/1
  [FResRr_N] -> Sum1/2
  Sum5/1 -> [mequiv_kg]
  [FDrag_N] -> Sum1/3
  [RRr_m] -> Square2/1
  [InRr_kgm2] -> Product7/1
  [InFr_kgm2] -> Product1/1
  Product7/1 -> Sum6/2
  [RFr_m] -> Square1/1
  [u0_mps] -> Delay1/2
  Delay1/1 -> [VgD_mps]
  [Vg_mps] -> Delay1/1
  [ax_mps2] -> Divide2/2
  [slipRr] -> Bus Creator4/2  "longSlip2"
  [slipFr] -> Bus Creator4/1  "longSlip1"
  [vWRr_mps] -> vWRr_mps/1  "vWRr_mps"
  [vWFr_mps] -> vWFr_mps/1  "vWFr_mps"
  [nWRr_RPM] -> nWRr_RPM/1  "nWRr_RPM"
  [nWFr_RPM] -> nWFr_RPM/1  "nWFr_RPM"
  [Vdist_m] -> Bus Creator5/8  "D_m"
  [Vg_mps] -> Bus Creator5/6  "Vg_mps"
  [ay_mps2] -> Bus Creator5/2  "ay_mps2"
  [slope_p] -> Divide/2
  slope%/1 -> [slope_p]
  InFr_kgm2/1 -> [InFr_kgm2]
  InRr_kgm2/1 -> [InRr_kgm2]
  RRr_m/1 -> [RRr_m]
  RFr_m/1 -> [RFr_m]
  FResRr_N/1 -> [FResRr_N]
  TMtrFr_Nm/1 -> [TMtrFr_Nm]
  TMtrRr_Nm/1 -> [TMtrRr_Nm]
  FResFr_N/1 -> [FResFr_N]
  Vspeed0_mps/1 -> [u0_mps]
  Subtract/1 -> Add1/1
  [ClRr] -> Divide9/2
  Divide9/1 -> Add1/2
  Divide1/1 -> Divide9/1, Divide8/2, Divide10/1
  [ClFr] -> Divide8/1
  Divide8/1 -> Add2/2
  Demux1/2 -> [ClRr]
  Demux1/1 -> [ClFr]
  Merge/1 -> Demux1/1
  Add1/1 -> [WRr_N]
  If Action Subsystem/1(Out1) -> Merge/2
  If Action Subsystem1/1 -> Merge/1
  If1/1 -> If Action Subsystem1/Action
  Mux3/1 -> If Action Subsystem1/1
  Constant24/1 -> Mux3/1
  Constant18/1 -> Mux3/2
  Mux1/1 -> If Action Subsystem/1(In1)
  [WTot_N] -> Divide13/2, Subtract/2
  Constant22/1 -> Divide2/1
  Constant21/1 -> Divide/1
  Constant10/1 -> Divide1/1
  Divide/1 -> Atan/1
  Constant16/1 -> Divide5/2
  Atan/1 -> Sin1/1, Sin/1
  Constant19/1 -> Divide5/1
  Sin1/1 -> Divide7/2
  Divide6/1 -> [FSlope_N]
  Sin/1 -> Divide6/2
  Divide7/1 -> [WTot_N]
  Divide5/1 -> Divide6/1, Divide7/1
  Constant17/1 -> Divide3/2
  Gain2/1 -> Divide13/1
  Constant13/1 -> Gain2/1
  Constant15/1 -> Divide3/1
  Add2/1 -> [WFr_N]
  Divide3/1 -> Divide4/2
  Square/1 -> Divide1/2
  Divide4/1 -> Add1/3, Add2/3
  If1/2 -> If Action Subsystem/Action
  [VgD_mps] -> Gain1/1
  Gain/1 -> Divide1/3
  Divide13/1 -> Add2/1, Subtract/1
  Constant23/1 -> If1/2
  Gain1/1 -> If1/1
  Divide2/1 -> Divide4/1
  density/1(rho) -> Gain/1
  [VgD_mps] -> Square/1
  [ax_mps2] -> Bus Creator5/1  "ax_mps2"
  delta_rad/1 -> [delta]
  [alpha1] -> Bus Creator4/3  "slipAngle1"
  [u_mps] -> Bus Creator5/3  "u_mps"
  [v_mps] -> Bus Creator5/4  "v_mps"
  [r_radps] -> Bus Creator5/5  "r_radps"
  [k_1pm] -> Bus Creator5/7  "k_1pm"
  Constant12/1 -> Product37/2
  Add13/1 -> [Fz_12]
  Sum12/1 -> Product23/1
  [Vg_mps] -> Discrete-Time Integrator2/1
  [TFrD_Nm] -> Sum22/1
  Sqrt/1 -> [Vg_mps]  "V_g"
  [v_mps] -> Product33/1
  [Vg_mps] -> Product31/2
  Constant25/1 -> Add25/2
  [Fy_21] -> Sum25/1
  [r_radps] -> Gain8/1
  [sin_delta] -> Product20/2
  [v_mps] -> Add12/1
  [Fy_11] -> Sum12/1
  [u_mps] -> Product28/2, Square3/1
  Rear Tires long/1 -> [miRr]  "miRr"
  [RRr_m] -> Product11/2
  Add10/1 -> Product15/1
  Product22/1 -> Sum14/1
  [Fy_12] -> Sum12/2
  [InFr_kgm2] -> Product40/1
  Gain18/1 -> Add7/2
  [slipRr] -> Rear Tires long/2
  [v_mps] -> Add10/1
  [u_mps] -> Add11/1
  Sum23/1 -> [vdot_mps2], Discrete-Time Integrator7/1
  [miFr] -> Product25/1
  [r_radps] -> Gain20/1
  [Fy_2] -> Sum11/1
  Product19/1 -> Sum10/1
  Demux2/1 -> [Fy_21]  "Fy_21"
  Demux2/2 -> [Fy_22]  "Fy_22"
  Sum14/1 -> Gain14/1
  [Fy_1] -> Product19/1
  Product24/1 -> Sum23/1
  [Fx_1t] -> Product20/1
  Product18/1 -> Sum23/2
  [u_mps] -> Product18/1
  Product25/1 -> [Fx_1]
  Product26/1 -> [Fx_2]
  [Fy_1] -> Product16/1
  Gain6/1 -> Add20/2
  [miRr] -> Product10/2
  Sum25/1 -> [Fy_2]
  [Fy_22] -> Sum25/2
  Atan5/1 -> [beta_rad]  "beta"
  [Fy_11] -> Sum26/1
  Gain19/1 -> Add10/2
  [sin_delta] -> Product16/2
  Gain5/1 -> Add20/1
  [Fz2] -> Product10/1
  Product16/1 -> Sum19/3
  [alpha_21] -> Mux5/1
  Sum10/1 -> Gain5/1, Sum11/2
  Product28/1 -> Atan5/1
  Discrete-Time Integrator/1 -> [u_mps]
  [v_mps] -> Product17/1
  [RFr_m] -> Product43/2
  Front Tires long/1 -> [miFr]  "miFr"
  Square3/1 -> Sum16/1
  [alpha_11] -> Mux4/1
  [Fz1] -> Front Tires long/1
  [RFr_m] -> Product21/1
  Atan4/1 -> Add25/1
  Atan2/1 -> Add5/1
  [Fz2] -> Rear Tires long/1
  Atan3/1 -> Add9/1
  [slipFr] -> Front Tires long/2
  Constant5/1 -> Add9/2
  Demux/1 -> [Fy_11]  "Fy_11"
  [Fy1] -> Demux/1
  Add9/1 -> [alpha_21]  "alpha_21"
  [u_mps] -> Add7/1
  [delta] -> Add5/2
  Add11/1 -> Product14/2
  [u_mps] -> Add24/1
  [alpha_22] -> Mux5/2
  Gain11/1 -> Add11/2
  Add3/1 -> [alpha_11]  "alpha_11"
  [v_mps] -> Add6/1
  Discrete-Time Integrator6/1 -> Product11/1, Gain4/1
  Constant6/1 -> Product27/1
  Atan1/1 -> Add3/1
  [cos_delta] -> Product22/2
  Gain20/1 -> Add24/2
  Product14/1 -> Atan4/1
  [r_radps] -> Gain19/1
  Product13/1 -> Atan1/1
  [cos_delta] -> Product/3
  Constant8/1 -> Product30/1
  Sum20/1 -> Product42/2
  [u_mps] -> Product34/2
  Constant9/1 -> Product36/1
  [delta] -> Add3/2
  [v_mps] -> Product28/1, Square4/1
  M1/1 -> Add18/2
  Add18/1 -> Product29/1
  [Fz1] -> Product25/2
  [r_radps] -> Product17/2
  Add20/1 -> Product27/2
  [r_radps] -> Gain18/1
  [Fy_12] -> Sum26/2
  Gain15/1 -> Add16/2, Add14/2
  Sum15/1 -> Gain13/1
  [u0_mps] -> Discrete-Time Integrator/2
  Sum17/1 -> [ay_mps2]  "a_y"
  [udot_mps2] -> Unit Delay1/1
  [Fz1] -> Product/2
  Gain9/1 -> Add8/2
  Discrete-Time Integrator2/1 -> [Vdist_m]
  Add8/1 -> Product12/1
  Gain8/1 -> Add4/2
  [r_radps] -> Gain7/1
  Product21/1 -> Sum22/2
  [RRr_m] -> Product44/2
  Product23/1 -> Sum14/2
  Product40/1 -> Discrete-Time Integrator3/1  "WFr_acc_rad/s"
  Sum21/1 -> Product41/1
  Add24/1 -> Product15/2
  [u_mps] -> Product44/1
  [InRr_kgm2] -> Product41/2
  Product41/1 -> Discrete-Time Integrator6/1  "WRr_acc_rad/s"
  Product44/1 -> Discrete-Time Integrator6/2
  [RFr_m] -> Product45/1
  Add7/1 -> Product12/2
  Sum19/1 -> Sum20/1
  [u_mps] -> Product43/1
  Product32/1 -> Sum21/1
  Product45/1 -> [vWFr_mps]
  Product11/1 -> [vWRr_mps]
  Gain4/1 -> [nWRr_RPM]
  Gain16/1 -> Discrete-Time Integrator9/1
  [vWFr_mps] -> Add19/1
  Add6/1 -> Product13/1
  [deWRr_N] -> Add16/1, Add14/1
  Product15/1 -> Atan3/1
  Product38/1 -> Add19/2
  [r_radps] -> Product34/1, Product33/2
  Sum26/1 -> [Fy_1]
  Product30/1 -> Product35/1, Product29/2
  Discrete-Time Integrator3/1 -> Product45/2, Gain3/1
  [r_radps] -> Gain9/1
  Product31/1 -> [k_1pm]  "curvature"
  [deWFr_N] -> Add15/2, Add13/2
  [Fz2] -> Product26/2
  Add19/1 -> Gain16/1
  Unit Delay3/1 -> Sum17/2
  Demux/2 -> [Fy_12]  "Fy_12"
  [r_radps] -> Gain10/1
  Product34/1 -> Sum17/1
  [v_mps] -> Add8/1
  Product33/1 -> Sum18/2
  [Fz_12] -> Mux6/2  "Fz_12"
  Gain13/1 -> Add20/4
  Constant3/1 -> Product24/1
  [FSlope_N] -> Sum20/3
  [r_radps] -> Product31/1
  [Fz_21] -> Mux7/1  "Fz_21"
  Mux6/1 -> [Fz1]  "Fz1_N"
  Product42/1 -> Sum24/1
  M3/1 -> Add18/1
  Constant7/1 -> Product42/1
  [miRr] -> Product26/1
  Gain12/1 -> Add15/1, Add13/1
  Add16/1 -> [Fz_21]
  [miFr] -> Product/1
  [sin_delta] -> Product23/2
  Product37/1 -> [deWRr_N]
  M2/1 -> Add17/1
  Product36/1 -> [deWFr_N]
  [r_radps] -> Gain11/1
  Gain10/1 -> Add12/2
  Sum18/1 -> [ax_mps2]  "a_x"
  Gain14/1 -> Add20/3
  Sum11/1 -> Product24/2
  [WRr_N] -> Gain15/1
  M4/1 -> Add17/2
  [FDrag_N] -> Sum20/2
  [r_radps] -> Product18/2
  [Fz_11] -> Mux6/1  "Fz_11"
  Product27/1 -> Discrete-Time Integrator8/1
  Discrete-Time Integrator8/1 -> [r_radps]  "r"
  Discrete-Time Integrator7/1 -> [v_mps]  "v"
  Gain3/1 -> [nWFr_RPM]
  Sum24/1 -> [udot_mps2], Discrete-Time Integrator/1
  Gain7/1 -> Add6/2
  [TRrD_Nm] -> Sum21/2
  [WFr_N] -> Gain12/1
  Square4/1 -> Sum16/2
  [u_mps] -> Add4/1
  Add14/1 -> [Fz_22]
  Product43/1 -> Discrete-Time Integrator3/2
  Add17/1 -> Product35/2
  Unit Delay1/1 -> Sum18/1
  Constant14/1 -> Add21/2
  Product20/1 -> Sum10/2
  Discrete-Time Integrator9/1 -> Add21/1, [slipFr]
  Product35/1 -> Product37/1
  Add4/1 -> Product13/2
  [cos_delta] -> Product19/2
  [vdot_mps2] -> Unit Delay3/1
  Add12/1 -> Product14/1
  Product29/1 -> Product36/2
  Product12/1 -> Atan2/1
  [Fz_22] -> Mux7/2  "Fz_22"
  [Fy_2] -> Gain6/1
  Sum13/1 -> Product22/1
  Add5/1 -> [alpha_12]  "alpha_12"
  [u_mps] -> Product38/1
  Add21/1 -> Product38/2
  Add15/1 -> [Fz_11]
  Sum16/1 -> Sqrt/1
  Sum22/1 -> Product40/2
  [alpha_12] -> Mux4/2
  Add25/1 -> [alpha_22]  "alpha_22"
  [ay_mps2] -> Product30/2
  Product17/1 -> Sum24/2
  [delta] -> Sin3/1, Sin2/1
  Sin3/1 -> [sin_delta]
  Sin2/1 -> [cos_delta]
  [alpha1] -> Front Tires lat/2
  [Fz1] -> Front Tires lat/1
  [Fz2] -> Rear Tires lat/1
  [alpha2] -> Rear Tires lat/2
  Mux4/1 -> [alpha1]
  Mux5/1 -> [alpha2]
  [Fy2] -> Demux2/1
  Bus Creator5/1 -> state/1
  [Fz2] -> Bus Creator/3  "Fz2_N"
  [alpha2] -> Bus Creator4/4  "slipAngle2"
  [Fx_1] -> Bus Creator/4  "Fx1_N"
  [Fx_2] -> Bus Creator/5  "Fx2_N"
  [Fy1] -> Bus Creator/6  "Fy1_N"
  [Fy2] -> Bus Creator/7  "Fy2_N"
  Bus Creator4/1 -> slip/1
  Mux7/1 -> [Fz2]  "Fz2_N"
  [Fz1] -> Bus Creator/2  "Fz1_N"
  [beta_rad] -> Bus Creator5/9  "beta_rad"
  Front Tires lat/1 -> Sum27/1
  Sum27/1 -> Discrete-Time Integrator11/1
  Discrete-Time Integrator11/1 -> Sum27/2, [Fy1]
  Discrete-Time Integrator12/1 -> [Fy2], Sum28/2
  Sum28/1 -> Discrete-Time Integrator12/1
  Rear Tires lat/1 -> Sum28/1
  Demux3/1 -> Sum13/1
  [Fx_1] -> Demux3/1
  Demux3/2 -> Sum13/2
  [Fx_2] -> Demux4/1
  Demux4/1 -> Sum15/1
  Demux4/2 -> Sum15/2
  Demux5/2 -> Sum29/2
  Demux5/1 -> Sum29/1
  [Fx_1] -> Demux5/1
  [Fx_2] -> Demux6/1
  Demux6/1 -> Sum30/1
  Demux6/2 -> Sum30/2
  Sum29/1 -> [Fx_1t]
  Sum30/1 -> [Fx_2t]
  Discrete-Time Integrator10/1 -> Add23/1, [slipRr]
  Add23/1 -> Product39/2
  Constant26/1 -> Add23/2
  Add22/1 -> Gain17/1
  Product39/1 -> Add22/2
  [vWRr_mps] -> Add22/1
  Gain17/1 -> Discrete-Time Integrator10/1
  [u_mps] -> Product39/1
  Product/1 -> Product21/2
  [FResFr_N] -> Sum19/2
  [FResRr_N] -> Sum19/4
  [Fx_1t] -> Sum19/1
  [Fx_2t] -> Sum19/5
  Product10/1 -> Product32/1
  [RRr_m] -> Product32/2

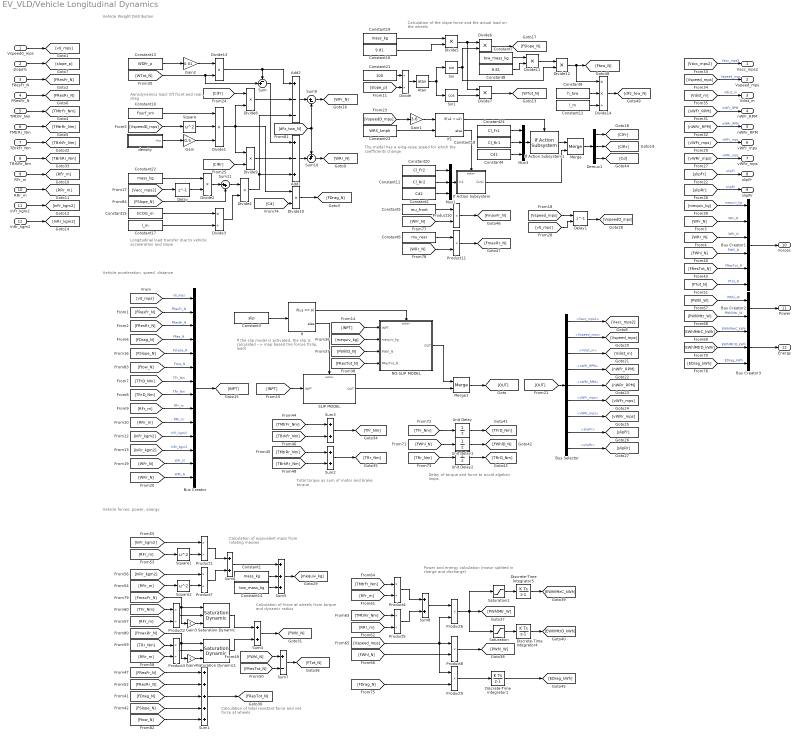
== system EV_VLD/Vehicle Longitudinal Dynamics ==
  note: Vehicle acceleration, speed, distance
  note: Vehicle Weight Distribution
  note: Vehicle forces, power, energy
  note: The model has a wing-raise speed for which the coefficients change
  note: Calculation of the slope force and the actual load on the wheels
  note: Aerodynamics load: lift front and rear, drag
  note: Longitudinal load transfer due to vehicle acceleration and slope
  note: If the slip model is activated, the slip is calculated --> map based tire forces f(slip, load)
  note: Total torque as sum of motor and brake torque
  note: Delay of torque and force to avoid algebric loops
  note: Calculation of equivalent mass from rotating masses
  note: Calculation of force at wheels from torque and dynamic radius
  note: Calculation of total resistant force and net force at wheels
  note: Power and energy calculation (motor splitted in charge and discharge)
  Vspeed0_mps : Inport
  slope% : Inport  Port=2
  FResFr_N : Inport  Port=3
  FResRr_N : Inport  Port=4
  TMtrFr_Nm : Inport  Port=5
  TMtrRr_Nm : Inport  Port=6
  TBrkFr_Nm : Inport  Port=7
  TBrkRr_Nm : Inport  Port=8
  RFr_m : Inport  Port=9
  RRr_m : Inport  Port=10
  InFr_kgm2 : Inport  Port=11
  InRr_kgm2 : Inport  Port=12
  Add1 : Sum  Inputs=+-+
  Add2 : Sum  Inputs=+--
  Atan : Trigonometry  Operator=atan
  Bus Creator : BusCreator  Inputs=14
  Bus Creator1 : BusCreator  Inputs=6
  Bus Creator2 : BusCreator  Inputs=2
  Bus Creator3 : BusCreator  Inputs=3
  Bus Selector : BusSelector  OutputSignals=Vacc_mps2,Vspeed_mps,Vdist_m,nWFr_RPM,nWRr_RPM,vWFr_mps,vWRr_mps,slipFr,slipRr
  Constant1 : Constant  Value=mass_kg
  Constant10 : Constant  Value=Fsurf_sm
  Constant11 : Constant  Value=Cl_Rr2
  Constant12 : Constant  Value=l_m
  Constant13 : Constant  Value=WDFr_p
  Constant14 : Constant  Value=tow_mass_kg
  Constant15 : Constant  Value=hCOG_m
  Constant16 : Constant  Value=9.81
  Constant17 : Constant  Value=l_m
  Constant18 : Constant  Value=Cl_Rr1
  Constant19 : Constant  Value=mass_kg
  Constant2 : Constant  Value=Cd2
  Constant20 : Constant  Value=Cl_Fr2
  Constant21 : Constant  Value=100
  Constant22 : Constant  Value=mass_kg
  Constant23 : Constant  Value=WRS_kmph
  Constant24 : Constant  Value=Cl_Fr1
  Constant3 : Constant  Value=slip
  Constant4 : Constant  Value=Cd1
  Constant5 : Constant  Value=mu_front
  Constant6 : Constant  Value=mu_rear
  Constant7 : Constant  Value=tow_mass_kg
  Constant8 : Constant  Value=9.81
  Constant9 : Constant  Value=h_tow
  Delay : Delay  DelayLength=1
  Delay1 : Delay  DelayLength=1  InitialConditionSource=Input port
      settings: InputPortMap=u0,p4
  Demux1 : Demux  Outputs=3
  Discrete-Time Integrator1 : DiscreteIntegrator  gainval=1e-3/3600  SampleTime=-1  ICPrevOutput=DiscIntNeverNeededParam  ICPrevScaledInput=DiscIntNeverNeededParam
  Discrete-Time Integrator4 : DiscreteIntegrator  gainval=1e-3/3600  SampleTime=-1  ICPrevOutput=DiscIntNeverNeededParam  ICPrevScaledInput=DiscIntNeverNeededParam
  Discrete-Time Integrator5 : DiscreteIntegrator  gainval=1e-3/3600  SampleTime=-1  ICPrevOutput=DiscIntNeverNeededParam  ICPrevScaledInput=DiscIntNeverNeededParam
  Divide : Product  Inputs=/*
  Divide1 : Product  Inputs=***
  Divide{2,4..13} (11 alike) : Product
  Divide14 : Product  Inputs=**/
  Divide3 : Product  Inputs=*/
  Gain : Gain  Gain=0.5
  Gain1 : Gain  Gain=3.6
  Gain2 : Gain  Gain=0.01
  Gain3 : Gain  Gain=-1
  Gain4 : Gain  Gain=-1
  If : If  IfExpression=u1 == 0
  If Action Subsystem : Subsystem  TreatAsAtomicUnit=on
  If Action Subsystem1 : $bdroot/Vehicle Longitudinal Dynamics/If Action Subsystem  SystemSampleTime=-1  Latency=0  AutoFrameSizeCalculation=off
  If1 : If  NumInputs=2  IfExpression=u1 < u2
  Merge : Merge
  Merge1 : Merge
  Mux1 : Mux  Inputs=3
  Mux3 : Mux  Inputs=3
  NO-SLIP MODEL : Subsystem  TreatAsAtomicUnit=on
  Product{1..5,7} (6 alike) : Product  Inputs=*/
  Product{6,8..11} (5 alike) : Product  Inputs=**
  SLIP MODEL : Subsystem  TreatAsAtomicUnit=on
  Saturation : Saturate  UpperLimit=inf  LowerLimit=0
  Saturation Dynamic : simulink/Discontinuities/Saturation Dynamic  OutMin=[]  OutMax=[]  OutDataTypeStr=Inherit: Same as second input  OutDataType=fixdt(1, 16)  OutScaling=2^-10  DoSatur=off
  Saturation Dynamic1 : simulink/Discontinuities/Saturation Dynamic  OutMin=[]  OutMax=[]  OutDataTypeStr=Inherit: Same as second input  OutDataType=fixdt(1, 16)  OutScaling=2^-10  DoSatur=off
  Saturation1 : Saturate  UpperLimit=0  LowerLimit=-inf
  Sin : Trigonometry
  Sin1 : Trigonometry  Operator=cos
  Square : Math  Operator=square  SignedPower=off  SaturateOnIntegerOverflow=on
  Square1 : Math  Operator=square  SignedPower=off  SaturateOnIntegerOverflow=on
  Square2 : Math  Operator=square  SignedPower=off  SaturateOnIntegerOverflow=on
  Sum : Sum  Inputs=-+|
  Sum1 : Sum  Inputs=+++++
  Sum10 : Sum  Inputs=++|
  Sum11 : Sum  Inputs=|++
  Sum{2..4,6,8} (5 alike) : Sum
  Sum5 : Sum  Inputs=+++
  Sum7 : Sum  Inputs=+-
  Sum9 : Sum  Inputs=|+-
  Unit Delay : UnitDelay  SampleTime=-1  HasFrameUpgradeWarning=on
  Unit Delay1 : UnitDelay  SampleTime=-1  HasFrameUpgradeWarning=on
  Unit Delay2 : UnitDelay  SampleTime=-1  HasFrameUpgradeWarning=on
  density : Subsystem
  Vacc_mps2 : Outport
  Vspeed_mps : Outport  Port=2
  Vdist_m : Outport  Port=3
  nWFr_RPM : Outport  Port=4
  nWRr_RPM : Outport  Port=5
  vWFr_mps : Outport  Port=6
  vWRr_mps : Outport  Port=7
  slipFr : Outport  Port=8
  slipRr : Outport  Port=9
  Forces : Outport  Port=10
  Power : Outport  Port=11
  Energy : Outport  Port=12
  wires:
  [VspeedD_mps] -> Square/1
  density/1(rho) -> Gain/1
  Gain1/1 -> If1/1
  Constant23/1 -> If1/2
  Divide13/1 -> Add2/1, Sum/1
  Gain/1 -> Divide1/3
  [VspeedD_mps] -> Gain1/1
  If1/2 -> If Action Subsystem/Action
  Divide4/1 -> Add2/3, Add1/3
  Square/1 -> Divide1/2
  Divide3/1 -> Divide4/2
  Constant15/1 -> Divide3/1
  Constant13/1 -> Gain2/1
  Gain2/1 -> Divide13/1
  Constant17/1 -> Divide3/2
  Divide5/1 -> Divide7/1, Divide6/1
  Divide7/1 -> [WTot_N]
  Sin/1 -> Divide12/2, Divide6/2
  Divide6/1 -> [FSlope_N]
  Sin1/1 -> Divide7/2
  Constant19/1 -> Divide5/1
  Atan/1 -> Sin/1, Sin1/1
  Constant16/1 -> Divide5/2
  Divide/1 -> Atan/1
  Constant10/1 -> Divide1/1
  Constant21/1 -> Divide/1
  Constant22/1 -> Divide2/1
  [Vacc_mps2] -> Delay/1
  [WTot_N] -> Sum/2, Divide13/2
  Mux1/1 -> If Action Subsystem/1(In1)
  Constant18/1 -> Mux3/2
  Constant24/1 -> Mux3/1
  Mux3/1 -> If Action Subsystem1/1
  If1/1 -> If Action Subsystem1/Action
  If Action Subsystem1/1 -> Merge/1
  If Action Subsystem/1(Out1) -> Merge/2
  Merge/1 -> Demux1/1
  Demux1/1 -> [ClFr]
  Demux1/2 -> [ClRr]
  Divide8/1 -> Add2/2
  [ClFr] -> Divide8/1
  Divide1/1 -> Divide10/1, Divide8/2, Divide9/1
  Divide9/1 -> Add1/2
  [ClRr] -> Divide9/2
  Sum/1 -> Add1/1
  Vspeed0_mps/1 -> [v0_mps]
  FResFr_N/1 -> [FResFr_N]
  TMtrRr_Nm/1 -> [TMtrRr_Nm]
  TMtrFr_Nm/1 -> [TMtrFr_Nm]
  FResRr_N/1 -> [FResRr_N]
  RFr_m/1 -> [RFr_m]
  RRr_m/1 -> [RRr_m]
  InRr_kgm2/1 -> [InRr_kgm2]
  InFr_kgm2/1 -> [InFr_kgm2]
  If/2 -> SLIP MODEL/Action
  If/1 -> NO-SLIP MODEL/Action
  [v0_mps] -> Bus Creator/1  "v0_mps"
  [FResFr_N] -> Bus Creator/2  "FResFr_N"
  [FResRr_N] -> Bus Creator/3  "FResRr_N"
  [FDrag_N] -> Bus Creator/4  "FRes_N"
  [TFrD_Nm] -> Bus Creator/7  "TFr_Nm"
  [TRrD_Nm] -> Bus Creator/8  "TRr_Nm"
  [RFr_m] -> Bus Creator/9  "RFr_m"
  [RRr_m] -> Bus Creator/10  "RRr_m"
  [InFr_kgm2] -> Bus Creator/11  "InFr_kgm2"
  [InRr_kgm2] -> Bus Creator/12  "InRr_kgm2"
  Bus Creator/1 -> [INPT]
  [INPT] -> NO-SLIP MODEL/1(INPT)
  [INPT] -> SLIP MODEL/1(INPT)
  Constant3/1 -> If/1
  NO-SLIP MODEL/1(OUT) -> Merge1/1
  SLIP MODEL/1(OUT) -> Merge1/2
  slope%/1 -> [slope_p]
  [slope_p] -> Divide/2
  [WFr_N] -> Bus Creator/13  "WFr_N"
  [WRr_N] -> Bus Creator/14  "WRr_N"
  Merge1/1 -> [OUT]
  [OUT] -> Bus Selector/1
  [Vacc_mps2] -> Vacc_mps2/1  "Vacc_mps2"
  [Vspeed_mps] -> Vspeed_mps/1  "Vspeed_mps"
  [Vdist_m] -> Vdist_m/1  "Vdist_m"
  [nWFr_RPM] -> nWFr_RPM/1  "nWFr_RPM"
  [nWRr_RPM] -> nWRr_RPM/1  "nWRr_RPM"
  [vWFr_mps] -> vWFr_mps/1  "vWFr_mps"
  [vWRr_mps] -> vWRr_mps/1  "vWRr_mps"
  [slipFr] -> slipFr/1  "slipFr"
  [slipRr] -> slipRr/1  "slipRr"
  [WFr_N] -> Bus Creator1/2  "WFr_N"
  [WRr_N] -> Bus Creator1/3  "WRr_N"
  Bus Selector/1 -> [Vacc_mps2]  "<Vacc_mps2>"
  Bus Selector/9 -> [slipRr]  "<slipRr>"
  Bus Selector/8 -> [slipFr]  "<slipFr>"
  Bus Selector/7 -> [vWRr_mps]  "<vWRr_mps>"
  Bus Selector/6 -> [vWFr_mps]  "<vWFr_mps>"
  Bus Selector/5 -> [nWRr_RPM]  "<nWRr_RPM>"
  Bus Selector/4 -> [nWFr_RPM]  "<nWFr_RPM>"
  Bus Selector/3 -> [Vdist_m]  "<Vdist_m>"
  Bus Selector/2 -> [Vspeed_mps]  "<Vspeed_mps>"
  Delay/1 -> Divide2/2
  [FSlope_N] -> Bus Creator/5  "Fslope_N"
  [Vspeed_mps] -> Delay1/1
  Delay1/1 -> [VspeedD_mps]
  [v0_mps] -> Delay1/2
  [RFr_m] -> Square1/1
  Product7/1 -> Sum6/2
  [InFr_kgm2] -> Product1/1
  [InRr_kgm2] -> Product7/1
  [RRr_m] -> Square2/1
  [FDrag_N] -> Sum1/3
  Sum5/1 -> [mequiv_kg]
  [FResRr_N] -> Sum1/2
  [FResFr_N] -> Sum1/1
  Product1/1 -> Sum6/1
  [RRr_m] -> Product3/2
  Sum4/1 -> [FWhl_N]
  Square2/1 -> Product7/2
  [RFr_m] -> Product2/2
  [TFr_Nm] -> Product2/1
  Sum1/1 -> [FResTot_N]
  [TRr_Nm] -> Product3/1
  Square1/1 -> Product1/2
  Sum6/1 -> Sum5/1
  [FSlope_N] -> Sum1/4
  [mequiv_kg] -> NO-SLIP MODEL/2(mequiv_kg)
  [FWhlD_N] -> NO-SLIP MODEL/3(FWhl_N)
  [FResTot_N] -> NO-SLIP MODEL/4(FResTot_N)
  [mequiv_kg] -> Bus Creator1/1  "mequiv_kg"
  [FWhl_N] -> Bus Creator1/4  "FWhl_N"
  [FResTot_N] -> Bus Creator1/5  "FResTot_N"
  Bus Creator1/1 -> Forces/1
  TBrkFr_Nm/1 -> [TBrkFr_Nm]
  TBrkRr_Nm/1 -> [TBrkRr_Nm]
  Sum3/1 -> [TFr_Nm]
  [TMtrFr_Nm] -> Sum3/1
  [TBrkFr_Nm] -> Sum3/2
  Sum2/1 -> [TRr_Nm]
  [TBrkRr_Nm] -> Sum2/2
  [TMtrRr_Nm] -> Sum2/1
  [FWhl_N] -> Sum7/1
  [FResTot_N] -> Sum7/2
  Sum7/1 -> [FTot_N]
  [FTot_N] -> Bus Creator1/6  "FTot_N"
  Bus Creator2/1 -> Power/1
  Product4/1 -> Sum8/1
  [TMtrRr_Nm] -> Product5/1
  Product5/1 -> Sum8/2
  [TMtrFr_Nm] -> Product4/1
  [RFr_m] -> Product4/2
  [RRr_m] -> Product5/2
  Sum8/1 -> Product6/1
  [Vspeed_mps] -> Product9/1, Product8/1, Product6/2
  Product6/1 -> Saturation1/1, Saturation/1, [PWhlMtr_W]
  [FWhl_N] -> Product8/2
  Product8/1 -> [PWhl_W]
  Discrete-Time Integrator5/1 -> [EWhlMtrC_kWh]
  Discrete-Time Integrator4/1 -> [EWhlMtrD_kWh]
  Saturation1/1 -> Discrete-Time Integrator5/1
  Saturation/1 -> Discrete-Time Integrator4/1
  [PWhl_W] -> Bus Creator2/1  "PWhl_W"
  [PWhlMtr_W] -> Bus Creator2/2  "PWhlMtr_W"
  [EWhlMtrD_kWh] -> Bus Creator3/2  "EWhlMtrD_kWh"
  [EWhlMtrC_kWh] -> Bus Creator3/1  "EWhlMtrC_kWh"
  Bus Creator3/1 -> Energy/1
  [TFr_Nm] -> Unit Delay/1
  [FWhl_N] -> Unit Delay1/1
  [TRr_Nm] -> Unit Delay2/1
  Unit Delay/1 -> [TFrD_Nm]
  Unit Delay1/1 -> [FWhlD_N]
  Unit Delay2/1 -> [TRrD_Nm]
  Constant4/1 -> Mux3/3
  Demux1/3 -> [Cd]
  Constant20/1 -> Mux1/1
  Constant11/1 -> Mux1/2
  Constant2/1 -> Mux1/3
  [Cd] -> Divide10/2
  Divide10/1 -> [FDrag_N]
  [FDrag_N] -> Product9/2
  Product9/1 -> Discrete-Time Integrator1/1
  Discrete-Time Integrator1/1 -> [EDrag_kWh]
  [EDrag_kWh] -> Bus Creator3/3  "EDrag_kWh"
  Product2/1 -> Saturation Dynamic/2
  Saturation Dynamic/1 -> Sum4/1
  Product3/1 -> Saturation Dynamic1/2
  Saturation Dynamic1/1 -> Sum4/2
  [WRr_N] -> Product11/2
  Constant5/1 -> Product10/1
  [WFr_N] -> Product10/2
  Constant6/1 -> Product11/1
  Product10/1 -> [FmaxFr_N]
  Product11/1 -> [FmaxRr_N]
  [FmaxFr_N] -> Saturation Dynamic/1, Gain3/1
  Gain3/1 -> Saturation Dynamic/3
  [FmaxRr_N] -> Saturation Dynamic1/1, Gain4/1
  Gain4/1 -> Saturation Dynamic1/3
  Constant7/1 -> Divide11/1
  Constant8/1 -> Divide11/2
  Divide11/1 -> Divide12/1
  Divide12/1 -> Divide14/1, [Ftow_N]
  Constant12/1 -> Divide14/3
  Constant9/1 -> Divide14/2
  Divide14/1 -> [dFz_tow_N]
  Sum9/1 -> [WFr_N]
  Add1/1 -> Sum10/2
  Sum10/1 -> [WRr_N]
  Add2/1 -> Sum9/1
  [dFz_tow_N] -> Sum10/1, Sum9/2
  Constant1/1 -> Sum5/2
  Constant14/1 -> Sum5/3
  [Ftow_N] -> Sum1/5
  [Ftow_N] -> Bus Creator/6  "Ftow_N"
  Divide2/1 -> Sum11/1
  Sum11/1 -> Divide4/1
  [FSlope_N] -> Sum11/2

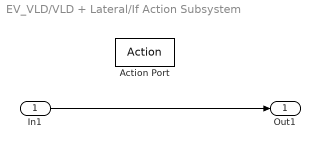
== system EV_VLD/VLD + Lateral/If Action Subsystem ==
  In1 : Inport
  Action Port : ActionPort
  Out1 : Outport
  wires:
  In1/1 -> Out1/1
